simulink model "case5"  (R2024b)
settings: Solver=FixedStepAuto  StartTime=0  StopTime=1  FixedStep=1e-7  RelTol=1e-3
values from neighbouring files (symbols this model uses):
  SG_D_1_D = 0.01056    [IEEE9_case_parameters.m]    (also in case1_parameters.m; case2_parameters.m; case3_parameters.m; case4_parameters.m)
  SG_D_1_EnableSaturation = 0    [IEEE9_case_parameters.m]    (also in case1_parameters.m; case2_parameters.m; case3_parameters.m; case4_parameters.m)
  SG_D_1_f0 = 60    [IEEE9_case_parameters.m]    (also in case1_parameters.m; case2_parameters.m; case3_parameters.m; case4_parameters.m)
  SG_D_1_H = 7.5    [IEEE9_case_parameters.m]    (also in case1_parameters.m; case2_parameters.m; case3_parameters.m; case4_parameters.m)
  SG_D_1_K_A = 20    [IEEE9_case_parameters.m]    (also in case1_parameters.m; case2_parameters.m; case3_parameters.m; case4_parameters.m)
  SG_D_1_K_E = 1.000000e+1    (= 10)    [IEEE9_case_parameters.m]    (also in case1_parameters.m; case2_parameters.m; case3_parameters.m; case4_parameters.m)
  SG_D_1_K_F = 2.363    [IEEE9_case_parameters.m]    (also in case1_parameters.m; case2_parameters.m; case3_parameters.m; case4_parameters.m)
  SG_D_1_K_s = 0.5    [IEEE9_case_parameters.m]    (also in case1_parameters.m = 5; case2_parameters.m = 5; case3_parameters.m = 5; case4_parameters.m = 5)
  SG_D_1_R_a = 0.001088    [IEEE9_case_parameters.m]    (also in case1_parameters.m; case2_parameters.m; case3_parameters.m; case4_parameters.m)
  SG_D_1_S_A = 1    [IEEE9_case_parameters.m]    (also in case1_parameters.m; case2_parameters.m; case3_parameters.m; case4_parameters.m)
  SG_D_1_S_B = 0.103    [IEEE9_case_parameters.m]    (also in case1_parameters.m; case2_parameters.m; case3_parameters.m; case4_parameters.m)
  SG_D_1_S_N = 10.659857    [IEEE9_case_parameters.m]    (also in case1_parameters.m; case2_parameters.m; case3_parameters.m; case4_parameters.m)
  SG_D_1_SpeedPara = 200    [IEEE9_case_parameters.m]    (also in case1_parameters.m; case2_parameters.m; case3_parameters.m; case4_parameters.m)
  SG_D_1_T_0 = 0.720173    [IEEE9_case_parameters.m]    (also in case1_parameters.m = 0.755522; case2_parameters.m = 0.808931; case3_parameters.m = 0.869402; case4_parameters.m = 0.729316)
  SG_D_1_T_1 = 0.3    [IEEE9_case_parameters.m]    (also in case1_parameters.m; case2_parameters.m; case3_parameters.m; case4_parameters.m)
  SG_D_1_T_2 = 0.05    [IEEE9_case_parameters.m]    (also in case1_parameters.m; case2_parameters.m; case3_parameters.m; case4_parameters.m)
  SG_D_1_T_3 = 0.02    [IEEE9_case_parameters.m]    (also in case1_parameters.m; case2_parameters.m; case3_parameters.m; case4_parameters.m)
  SG_D_1_T_4 = 0.005    [IEEE9_case_parameters.m]    (also in case1_parameters.m; case2_parameters.m; case3_parameters.m; case4_parameters.m)
  SG_D_1_T_A = 0.02    [IEEE9_case_parameters.m]    (also in case1_parameters.m; case2_parameters.m; case3_parameters.m; case4_parameters.m)
  SG_D_1_T_dd = 8.000000e+0    (= 8)    [IEEE9_case_parameters.m]    (also in case1_parameters.m; case2_parameters.m; case3_parameters.m; case4_parameters.m)
  SG_D_1_T_ddd = 0.04    [IEEE9_case_parameters.m]    (also in case1_parameters.m; case2_parameters.m; case3_parameters.m; case4_parameters.m)
  SG_D_1_T_E = 0.314    [IEEE9_case_parameters.m]    (also in case1_parameters.m; case2_parameters.m; case3_parameters.m; case4_parameters.m)
  SG_D_1_T_F = 0.35    [IEEE9_case_parameters.m]    (also in case1_parameters.m; case2_parameters.m; case3_parameters.m; case4_parameters.m)
  SG_D_1_T_qd = 0.8    [IEEE9_case_parameters.m]    (also in case1_parameters.m; case2_parameters.m; case3_parameters.m; case4_parameters.m)
  SG_D_1_T_qdd = 0.02    [IEEE9_case_parameters.m]    (also in case1_parameters.m; case2_parameters.m; case3_parameters.m; case4_parameters.m)
  SG_D_1_T_speed = 0.1    [IEEE9_case_parameters.m]    (also in case1_parameters.m = 200; case2_parameters.m = 200; case3_parameters.m = 200; case4_parameters.m = 200)
  SG_D_1_T_w = 0.5    [IEEE9_case_parameters.m]    (also in case1_parameters.m; case2_parameters.m; case3_parameters.m; case4_parameters.m)
  SG_D_1_V_ref = 1.990276    [IEEE9_case_parameters.m]    (also in case1_parameters.m = 2.042296; case2_parameters.m = 2.051388; case3_parameters.m = 2.089584; case4_parameters.m = 2.01845)
  SG_D_1_w_ref = 376.991118    [IEEE9_case_parameters.m]    (also in case1_parameters.m; case2_parameters.m; case3_parameters.m; case4_parameters.m)
  SG_D_1_wb = 6.000000e+1    (= 60)    [IEEE9_case_parameters.m]    (also in case1_parameters.m; case2_parameters.m; case3_parameters.m; case4_parameters.m)
  SG_D_1_x_d = 1.9    [IEEE9_case_parameters.m]    (also in case1_parameters.m; case2_parameters.m; case3_parameters.m; case4_parameters.m)
  SG_D_1_x_dd = 0.302    [IEEE9_case_parameters.m]    (also in case1_parameters.m; case2_parameters.m; case3_parameters.m; case4_parameters.m)
  SG_D_1_x_ddd = 0.204    [IEEE9_case_parameters.m]    (also in case1_parameters.m; case2_parameters.m; case3_parameters.m; case4_parameters.m)
  SG_D_1_x_l = 0.05    [IEEE9_case_parameters.m]    (also in case1_parameters.m; case2_parameters.m; case3_parameters.m; case4_parameters.m)
  SG_D_1_x_q = 1.3    [IEEE9_case_parameters.m]    (also in case1_parameters.m; case2_parameters.m; case3_parameters.m; case4_parameters.m)
  SG_D_1_x_qd = 0.5    [IEEE9_case_parameters.m]    (also in case1_parameters.m; case2_parameters.m; case3_parameters.m; case4_parameters.m)
  SG_D_1_x_qdd = 0.3    [IEEE9_case_parameters.m]    (also in case1_parameters.m; case2_parameters.m; case3_parameters.m; case4_parameters.m)
  SG_D_2_D = 0.02    [IEEE9_case_parameters.m]    (also in case1_parameters.m; case2_parameters.m; case3_parameters.m; case4_parameters.m)
  SG_D_2_EnableSaturation = 0    [IEEE9_case_parameters.m]    (also in case1_parameters.m; case2_parameters.m; case3_parameters.m; case4_parameters.m)
  SG_D_2_f0 = 60    [IEEE9_case_parameters.m]    (also in case1_parameters.m; case2_parameters.m; case3_parameters.m; case4_parameters.m)
  SG_D_2_H = 8.000000e+0    (= 8)    [IEEE9_case_parameters.m]    (also in case1_parameters.m; case2_parameters.m; case3_parameters.m; case4_parameters.m)
  SG_D_2_K_A = 20    [IEEE9_case_parameters.m]    (also in case1_parameters.m; case2_parameters.m; case3_parameters.m; case4_parameters.m)
  SG_D_2_K_E = 1.000000e+1    (= 10)    [IEEE9_case_parameters.m]    (also in case1_parameters.m; case2_parameters.m; case3_parameters.m; case4_parameters.m)
  SG_D_2_K_F = 2.363    [IEEE9_case_parameters.m]    (also in case1_parameters.m; case2_parameters.m; case3_parameters.m; case4_parameters.m)
  SG_D_2_K_s = 0.5    [IEEE9_case_parameters.m]    (also in case1_parameters.m = 4; case2_parameters.m = 4; case3_parameters.m = 4; case4_parameters.m = 4)
  SG_D_2_R_a = 0.001088    [IEEE9_case_parameters.m]    (also in case1_parameters.m; case2_parameters.m; case3_parameters.m; case4_parameters.m)
  SG_D_2_S_A = 1    [IEEE9_case_parameters.m]    (also in case1_parameters.m; case2_parameters.m; case3_parameters.m; case4_parameters.m)
  SG_D_2_S_B = 0.103    [IEEE9_case_parameters.m]    (also in case1_parameters.m; case2_parameters.m; case3_parameters.m; case4_parameters.m)
  SG_D_2_S_N = 10.659857    [IEEE9_case_parameters.m]    (also in case1_parameters.m; case2_parameters.m; case3_parameters.m; case4_parameters.m)
  SG_D_2_SpeedPara = 200    [IEEE9_case_parameters.m]    (also in case1_parameters.m; case2_parameters.m; case3_parameters.m; case4_parameters.m)
  SG_D_2_T_0 = 1.632913    [IEEE9_case_parameters.m]    (also in case1_parameters.m = 1.632925; case2_parameters.m = 1.632915; case3_parameters.m = 1.632914; case4_parameters.m = 1.632927)
  SG_D_2_T_1 = 0.2    [IEEE9_case_parameters.m]    (also in case1_parameters.m; case2_parameters.m; case3_parameters.m; case4_parameters.m)
  SG_D_2_T_2 = 0.05    [IEEE9_case_parameters.m]    (also in case1_parameters.m; case2_parameters.m; case3_parameters.m; case4_parameters.m)
  SG_D_2_T_3 = 0.02    [IEEE9_case_parameters.m]    (also in case1_parameters.m; case2_parameters.m; case3_parameters.m; case4_parameters.m)
  SG_D_2_T_4 = 0.005    [IEEE9_case_parameters.m]    (also in case1_parameters.m; case2_parameters.m; case3_parameters.m; case4_parameters.m)
  SG_D_2_T_A = 0.02    [IEEE9_case_parameters.m]    (also in case1_parameters.m; case2_parameters.m; case3_parameters.m; case4_parameters.m)
  SG_D_2_T_dd = 7.9    [IEEE9_case_parameters.m]    (also in case1_parameters.m; case2_parameters.m; case3_parameters.m; case4_parameters.m)
  SG_D_2_T_ddd = 0.04    [IEEE9_case_parameters.m]    (also in case1_parameters.m; case2_parameters.m; case3_parameters.m; case4_parameters.m)
  SG_D_2_T_E = 0.314    [IEEE9_case_parameters.m]    (also in case1_parameters.m; case2_parameters.m; case3_parameters.m; case4_parameters.m)
  SG_D_2_T_F = 0.35    [IEEE9_case_parameters.m]    (also in case1_parameters.m; case2_parameters.m; case3_parameters.m; case4_parameters.m)
  SG_D_2_T_qd = 0.8    [IEEE9_case_parameters.m]    (also in case1_parameters.m; case2_parameters.m; case3_parameters.m; case4_parameters.m)
  SG_D_2_T_qdd = 0.015    [IEEE9_case_parameters.m]    (also in case1_parameters.m; case2_parameters.m; case3_parameters.m; case4_parameters.m)
  SG_D_2_T_speed = 0.1    [IEEE9_case_parameters.m]    (also in case1_parameters.m = 150; case2_parameters.m = 150; case3_parameters.m = 150; case4_parameters.m = 150)
  SG_D_2_T_w = 0.35    [IEEE9_case_parameters.m]    (also in case1_parameters.m; case2_parameters.m; case3_parameters.m; case4_parameters.m)
  SG_D_2_V_ref = 2.58547    [IEEE9_case_parameters.m]    (also in case1_parameters.m = 2.597896; case2_parameters.m = 2.587136; case3_parameters.m = 2.586042; case4_parameters.m = 2.599679)
  SG_D_2_w_ref = 376.991118    [IEEE9_case_parameters.m]    (also in case1_parameters.m; case2_parameters.m; case3_parameters.m; case4_parameters.m)
  SG_D_2_wb = 6.000000e+1    (= 60)    [IEEE9_case_parameters.m]    (also in case1_parameters.m; case2_parameters.m; case3_parameters.m; case4_parameters.m)
  SG_D_2_x_d = 1.8    [IEEE9_case_parameters.m]    (also in case1_parameters.m; case2_parameters.m; case3_parameters.m; case4_parameters.m)
  SG_D_2_x_dd = 0.302    [IEEE9_case_parameters.m]    (also in case1_parameters.m; case2_parameters.m; case3_parameters.m; case4_parameters.m)
  SG_D_2_x_ddd = 0.204    [IEEE9_case_parameters.m]    (also in case1_parameters.m; case2_parameters.m; case3_parameters.m; case4_parameters.m)
  SG_D_2_x_l = 0.05    [IEEE9_case_parameters.m]    (also in case1_parameters.m; case2_parameters.m; case3_parameters.m; case4_parameters.m)
  SG_D_2_x_q = 1.25    [IEEE9_case_parameters.m]    (also in case1_parameters.m; case2_parameters.m; case3_parameters.m; case4_parameters.m)
  SG_D_2_x_qd = 0.5    [IEEE9_case_parameters.m]    (also in case1_parameters.m; case2_parameters.m; case3_parameters.m; case4_parameters.m)
  SG_D_2_x_qdd = 0.3    [IEEE9_case_parameters.m]    (also in case1_parameters.m; case2_parameters.m; case3_parameters.m; case4_parameters.m)
  SG_D_3_D = 0.02    [IEEE9_case_parameters.m]    (also in case1_parameters.m; case2_parameters.m; case3_parameters.m; case4_parameters.m)
  SG_D_3_EnableSaturation = 0    [IEEE9_case_parameters.m]    (also in case1_parameters.m; case2_parameters.m; case3_parameters.m; case4_parameters.m)
  SG_D_3_f0 = 60    [IEEE9_case_parameters.m]    (also in case1_parameters.m; case2_parameters.m; case3_parameters.m; case4_parameters.m)
  SG_D_3_H = 7.7    [IEEE9_case_parameters.m]    (also in case1_parameters.m; case2_parameters.m; case3_parameters.m; case4_parameters.m)
  SG_D_3_K_A = 20    [IEEE9_case_parameters.m]    (also in case1_parameters.m; case2_parameters.m; case3_parameters.m; case4_parameters.m)
  SG_D_3_K_E = 1.000000e+1    (= 10)    [IEEE9_case_parameters.m]    (also in case1_parameters.m; case2_parameters.m; case3_parameters.m; case4_parameters.m)
  SG_D_3_K_F = 2.363    [IEEE9_case_parameters.m]    (also in case1_parameters.m; case2_parameters.m; case3_parameters.m; case4_parameters.m)
  SG_D_3_K_s = 0.2    [IEEE9_case_parameters.m]    (also in case1_parameters.m = 2; case2_parameters.m = 2; case3_parameters.m = 2; case4_parameters.m = 2)
  SG_D_3_R_a = 0.001088    [IEEE9_case_parameters.m]    (also in case1_parameters.m; case2_parameters.m; case3_parameters.m; case4_parameters.m)
  SG_D_3_S_A = 1    [IEEE9_case_parameters.m]    (also in case1_parameters.m; case2_parameters.m; case3_parameters.m; case4_parameters.m)
  SG_D_3_S_B = 0.103    [IEEE9_case_parameters.m]    (also in case1_parameters.m; case2_parameters.m; case3_parameters.m; case4_parameters.m)
  SG_D_3_S_N = 10.659857    [IEEE9_case_parameters.m]    (also in case1_parameters.m; case2_parameters.m; case3_parameters.m; case4_parameters.m)
  SG_D_3_SpeedPara = 200    [IEEE9_case_parameters.m]    (also in case1_parameters.m; case2_parameters.m; case3_parameters.m; case4_parameters.m)
  SG_D_3_T_0 = 0.850788    [IEEE9_case_parameters.m]    (also in case1_parameters.m = 0.850786; case2_parameters.m = 0.850787; case3_parameters.m; case4_parameters.m = 0.850786)
  SG_D_3_T_1 = 0.2    [IEEE9_case_parameters.m]    (also in case1_parameters.m; case2_parameters.m; case3_parameters.m; case4_parameters.m)
  SG_D_3_T_2 = 0.05    [IEEE9_case_parameters.m]    (also in case1_parameters.m; case2_parameters.m; case3_parameters.m; case4_parameters.m)
  SG_D_3_T_3 = 0.02    [IEEE9_case_parameters.m]    (also in case1_parameters.m; case2_parameters.m; case3_parameters.m; case4_parameters.m)
  SG_D_3_T_4 = 0.005    [IEEE9_case_parameters.m]    (also in case1_parameters.m; case2_parameters.m; case3_parameters.m; case4_parameters.m)
  SG_D_3_T_A = 0.02    [IEEE9_case_parameters.m]    (also in case1_parameters.m; case2_parameters.m; case3_parameters.m; case4_parameters.m)
  SG_D_3_T_dd = 8.1    [IEEE9_case_parameters.m]    (also in case1_parameters.m; case2_parameters.m; case3_parameters.m; case4_parameters.m)
  SG_D_3_T_ddd = 0.04    [IEEE9_case_parameters.m]    (also in case1_parameters.m; case2_parameters.m; case3_parameters.m; case4_parameters.m)
  SG_D_3_T_E = 0.314    [IEEE9_case_parameters.m]    (also in case1_parameters.m; case2_parameters.m; case3_parameters.m; case4_parameters.m)
  SG_D_3_T_F = 0.35    [IEEE9_case_parameters.m]    (also in case1_parameters.m; case2_parameters.m; case3_parameters.m; case4_parameters.m)
  SG_D_3_T_qd = 0.8    [IEEE9_case_parameters.m]    (also in case1_parameters.m; case2_parameters.m; case3_parameters.m; case4_parameters.m)
  SG_D_3_T_qdd = 0.015    [IEEE9_case_parameters.m]    (also in case1_parameters.m; case2_parameters.m; case3_parameters.m; case4_parameters.m)
  SG_D_3_T_speed = 0.1    [IEEE9_case_parameters.m]    (also in case1_parameters.m = 180; case2_parameters.m = 180; case3_parameters.m = 180; case4_parameters.m = 180)
  SG_D_3_T_w = 0.4    [IEEE9_case_parameters.m]    (also in case1_parameters.m; case2_parameters.m; case3_parameters.m; case4_parameters.m)
  SG_D_3_V_ref = 1.892727    [IEEE9_case_parameters.m]    (also in case1_parameters.m = 1.906439; case2_parameters.m = 1.895535; case3_parameters.m = 1.892105; case4_parameters.m = 1.906598)
  SG_D_3_w_ref = 376.991118    [IEEE9_case_parameters.m]    (also in case1_parameters.m; case2_parameters.m; case3_parameters.m; case4_parameters.m)
  SG_D_3_wb = 6.000000e+1    (= 60)    [IEEE9_case_parameters.m]    (also in case1_parameters.m; case2_parameters.m; case3_parameters.m; case4_parameters.m)
  SG_D_3_x_d = 1.85    [IEEE9_case_parameters.m]    (also in case1_parameters.m; case2_parameters.m; case3_parameters.m; case4_parameters.m)
  SG_D_3_x_dd = 0.302    [IEEE9_case_parameters.m]    (also in case1_parameters.m; case2_parameters.m; case3_parameters.m; case4_parameters.m)
  SG_D_3_x_ddd = 0.204    [IEEE9_case_parameters.m]    (also in case1_parameters.m; case2_parameters.m; case3_parameters.m; case4_parameters.m)
  SG_D_3_x_l = 0.05    [IEEE9_case_parameters.m]    (also in case1_parameters.m; case2_parameters.m; case3_parameters.m; case4_parameters.m)
  SG_D_3_x_q = 1.2    [IEEE9_case_parameters.m]    (also in case1_parameters.m; case2_parameters.m; case3_parameters.m; case4_parameters.m)
  SG_D_3_x_qd = 0.5    [IEEE9_case_parameters.m]    (also in case1_parameters.m; case2_parameters.m; case3_parameters.m; case4_parameters.m)
  SG_D_3_x_qdd = 0.3    [IEEE9_case_parameters.m]    (also in case1_parameters.m; case2_parameters.m; case3_parameters.m; case4_parameters.m)
(part 9 of 12)

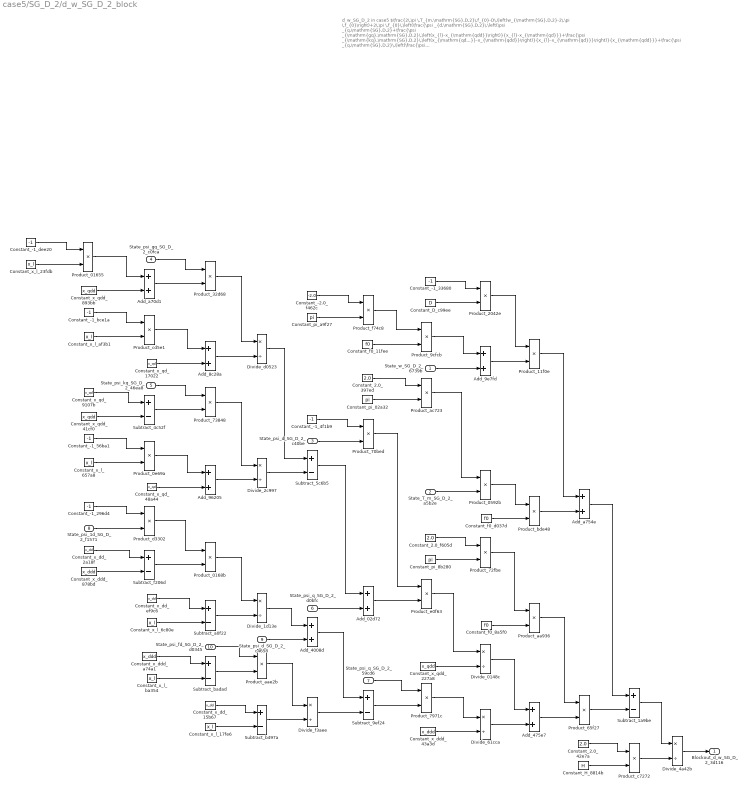
== system case5/SG_D_2/d_w_SG_D_2_block ==
  note: d_w_SG_D_2 in case5
      | $\frac{2\,\pi \,T_{m,\mathrm{SG},D,2}\,f_{0}-D\,\left(w_{\mathrm{SG},D,2}-2\,\pi \,f_{0}\right)+2\,\pi \,f_{0}\,\left(\frac{\psi _{d,\mathrm{SG},D,2}\,\left(\psi _{q,\mathrm{SG},D,2}+\frac{\psi _{\mathrm{gq},\mathrm{SG},D,2}\,\left(x_{l}-x_{\mathrm{qdd}}\right)}{x_{l}-x_{\mathrm{qd}}}+\frac{\psi _{\mathrm{kq},\mathrm{SG},D,2}\,\left(x_{\mathrm{qd}}-x_{\mathrm{qdd}}\right)}{x_{l}-x_{\mathrm{qd}}}\right)}{x_{\mathrm{qdd}}}+\frac{\psi _{q,\mathrm{SG},D,2}\,\left(\frac{\psi _{\mathrm{1d},\mathrm{SG},D,2}\,\left(x_{\mathrm{dd}}-x_{\mathrm{ddd}}\right)}{x_{\mathrm{dd}}-x_{l}}-\psi _{d,\mathrm{SG},D,2}+\frac{\psi _{\mathrm{fd},\mathrm{SG},D,2}\,\left(x_{\mathrm{ddd}}-x_{l}\right)}{x_{\mathrm{dd}}-x_{l}}\right)}{x_{\mathrm{ddd}}}\right)}{2\,H}$
      | Automatically generated on 2025-10-31 19:11:25 .
  State_w_SG_D_2_6739b : Inport
  State_T_m_SG_D_2_a5b2e : Inport  Port=2
  State_psi_d_SG_D_2_c40be : Inport  Port=3
  State_psi_gq_SG_D_2_c0fca : Inport  Port=4
  State_psi_kq_SG_D_2_46ea8 : Inport  Port=5
  State_psi_q_SG_D_2_d0bfc : Inport  Port=6
  State_psi_q_SG_D_2_59cd6 : Inport  Port=7
  State_psi_1d_SG_D_2_f1571 : Inport  Port=8
  State_psi_d_SG_D_2_c4658 : Inport  Port=9
  State_psi_fd_SG_D_2_d0345 : Inport  Port=10
  Add_02d72 : Sum
  Add_4008d : Sum
  Add_475e7 : Sum
  Add_8c28a : Sum
  Add_96205 : Sum
  Add_9e7fd : Sum
  Add_a70d1 : Sum
  Add_a754e : Sum
  Constant_-1_296d4 : Constant  Value=-1
  Constant_-1_33680 : Constant  Value=-1
  Constant_-1_4f1b9 : Constant  Value=-1
  Constant_-1_56ba1 : Constant  Value=-1
  Constant_-1_bce1a : Constant  Value=-1
  Constant_-1_dee20 : Constant  Value=-1
  Constant_-2.0_f462c : Constant  Value=-2.0
  Constant_2.0_397ed : Constant  Value=2.0
  Constant_2.0_42e7a : Constant  Value=2.0
  Constant_2.0_f605d : Constant  Value=2.0
  Constant_D_c99ee : Constant  Value=D
  Constant_H_8814b : Constant  Value=H
  Constant_f0_11fee : Constant  Value=f0
  Constant_f0_8a5f0 : Constant  Value=f0
  Constant_f0_d037d : Constant  Value=f0
  Constant_pi_02a32 : Constant  Value=pi
  Constant_pi_8b280 : Constant  Value=pi
  Constant_pi_a9f27 : Constant  Value=pi
  Constant_x_dd_15b67 : Constant  Value=x_dd
  Constant_x_dd_2a18f : Constant  Value=x_dd
  Constant_x_dd_ef9c6 : Constant  Value=x_dd
  Constant_x_ddd_43a3d : Constant  Value=x_ddd
  Constant_x_ddd_878bd : Constant  Value=x_ddd
  Constant_x_ddd_a74a1 : Constant  Value=x_ddd
  Constant_x_l_17fe6 : Constant  Value=x_l
  Constant_x_l_23fdb : Constant  Value=x_l
  Constant_x_l_657a8 : Constant  Value=x_l
  Constant_x_l_6c80e : Constant  Value=x_l
  Constant_x_l_af3b1 : Constant  Value=x_l
  Constant_x_l_ba354 : Constant  Value=x_l
  Constant_x_qd_17022 : Constant  Value=x_qd
  Constant_x_qd_48a44 : Constant  Value=x_qd
  Constant_x_qd_9107b : Constant  Value=x_qd
  Constant_x_qdd_227a8 : Constant  Value=x_qdd
  Constant_x_qdd_41cf0 : Constant  Value=x_qdd
  Constant_x_qdd_893bb : Constant  Value=x_qdd
  Divide_0148c : Product  Inputs=*/
  Divide_1d13e : Product  Inputs=*/
  Divide_2c997 : Product  Inputs=*/
  Divide_4a42b : Product  Inputs=*/
  Divide_61cca : Product  Inputs=*/
  Divide_d0523 : Product  Inputs=*/
  Divide_f3aee : Product  Inputs=*/
  Product_01655 : Product
  Product_0168b : Product
  Product_0592b : Product
  Product_0e69a : Product
  Product_11f0e : Product
  Product_2042e : Product
  Product_32d68 : Product
  Product_65f27 : Product
  Product_70bed : Product
  Product_72fbe : Product
  Product_73848 : Product
  Product_7971c : Product
  Product_9cfcb : Product
  Product_aa936 : Product
  Product_aae2b : Product
  Product_ac723 : Product
  Product_bde48 : Product
  Product_c7272 : Product
  Product_cd5e1 : Product
  Product_d3302 : Product
  Product_e0f63 : Product
  Product_f74c8 : Product
  Subtract_1a9be : Sum  Inputs=+-
  Subtract_4c52f : Sum  Inputs=+-
  Subtract_5c6b5 : Sum  Inputs=+-
  Subtract_9ef24 : Sum  Inputs=+-
  Subtract_a0f22 : Sum  Inputs=+-
  Subtract_b497a : Sum  Inputs=+-
  Subtract_badad : Sum  Inputs=+-
  Subtract_f206d : Sum  Inputs=+-
  Blockout_d_w_SG_D_2_3d116 : Outport
  wires:
  Constant_x_qd_9107b/1 -> Subtract_4c52f/1
  Constant_-1_56ba1/1 -> Product_0e69a/1
  Constant_-1_dee20/1 -> Product_01655/1
  Constant_x_qdd_41cf0/1 -> Subtract_4c52f/2
  Subtract_b497a/1 -> Divide_f3aee/2
  Constant_x_l_657a8/1 -> Product_0e69a/2
  Constant_x_l_23fdb/1 -> Product_01655/2
  Product_0e69a/1 -> Add_96205/1
  Product_01655/1 -> Add_a70d1/1
  Constant_x_l_6c80e/1 -> Subtract_a0f22/2
  Constant_x_l_af3b1/1 -> Product_cd5e1/2
  Constant_x_ddd_43a3d/1 -> Divide_61cca/2
  Subtract_badad/1 -> Product_aae2b/2
  Constant_x_qd_48a44/1 -> Add_96205/2
  Constant_x_qdd_893bb/1 -> Add_a70d1/2
  Constant_-1_bce1a/1 -> Product_cd5e1/1
  State_psi_d_SG_D_2_c40be/1 -> Product_70bed/2
  Constant_-1_296d4/1 -> Product_d3302/1
  State_w_SG_D_2_6739b/1 -> Add_9e7fd/2
  Product_cd5e1/1 -> Add_8c28a/1
  State_psi_1d_SG_D_2_f1571/1 -> Product_d3302/2
  Constant_x_dd_2a18f/1 -> Subtract_f206d/1
  Divide_d0523/1 -> Subtract_5c6b5/1
  Subtract_4c52f/1 -> Product_73848/2
  Constant_x_ddd_878bd/1 -> Subtract_f206d/2
  State_psi_gq_SG_D_2_c0fca/1 -> Product_32d68/1
  Add_96205/1 -> Divide_2c997/2
  State_psi_d_SG_D_2_c4658/1 -> Add_4008d/2
  Add_a70d1/1 -> Product_32d68/2
  Constant_x_qd_17022/1 -> Add_8c28a/2
  State_psi_kq_SG_D_2_46ea8/1 -> Product_73848/1
  Product_d3302/1 -> Product_0168b/1
  Subtract_f206d/1 -> Product_0168b/2
  Constant_pi_02a32/1 -> Product_ac723/2
  Constant_x_dd_ef9c6/1 -> Subtract_a0f22/1
  Constant_x_ddd_a74a1/1 -> Subtract_badad/1
  Constant_x_l_ba354/1 -> Subtract_badad/2
  Product_32d68/1 -> Divide_d0523/1
  Add_8c28a/1 -> Divide_d0523/2
  Add_02d72/1 -> Product_e0f63/2
  Product_73848/1 -> Divide_2c997/1
  Constant_pi_a9f27/1 -> Product_f74c8/2
  Product_0168b/1 -> Divide_1d13e/1
  Subtract_a0f22/1 -> Divide_1d13e/2
  State_psi_fd_SG_D_2_d0345/1 -> Product_aae2b/1
  Divide_1d13e/1 -> Add_4008d/1
  Constant_x_dd_15b67/1 -> Subtract_b497a/1
  Constant_x_l_17fe6/1 -> Subtract_b497a/2
  Divide_2c997/1 -> Subtract_5c6b5/2
  Product_aae2b/1 -> Divide_f3aee/1
  Constant_-1_4f1b9/1 -> Product_70bed/1
  Constant_-2.0_f462c/1 -> Product_f74c8/1
  Subtract_5c6b5/1 -> Add_02d72/1
  Subtract_9ef24/1 -> Product_7971c/2
  State_psi_q_SG_D_2_d0bfc/1 -> Add_02d72/2
  Constant_D_c99ee/1 -> Product_2042e/2
  Add_4008d/1 -> Subtract_9ef24/1
  Divide_f3aee/1 -> Subtract_9ef24/2
  Product_f74c8/1 -> Product_9cfcb/1
  Constant_f0_11fee/1 -> Product_9cfcb/2
  Constant_2.0_397ed/1 -> Product_ac723/1
  Product_70bed/1 -> Product_e0f63/1
  State_psi_q_SG_D_2_59cd6/1 -> Product_7971c/1
  Constant_-1_33680/1 -> Product_2042e/1
  Product_9cfcb/1 -> Add_9e7fd/1
  Product_ac723/1 -> Product_0592b/1
  State_T_m_SG_D_2_a5b2e/1 -> Product_0592b/2
  Constant_2.0_f605d/1 -> Product_72fbe/1
  Constant_pi_8b280/1 -> Product_72fbe/2
  Product_e0f63/1 -> Divide_0148c/1
  Constant_x_qdd_227a8/1 -> Divide_0148c/2
  Product_7971c/1 -> Divide_61cca/1
  Product_2042e/1 -> Product_11f0e/1
  Add_9e7fd/1 -> Product_11f0e/2
  Product_0592b/1 -> Product_bde48/1
  Constant_f0_d037d/1 -> Product_bde48/2
  Product_72fbe/1 -> Product_aa936/1
  Constant_f0_8a5f0/1 -> Product_aa936/2
  Divide_0148c/1 -> Add_475e7/1
  Divide_61cca/1 -> Add_475e7/2
  Product_11f0e/1 -> Add_a754e/1
  Product_bde48/1 -> Add_a754e/2
  Product_aa936/1 -> Product_65f27/1
  Add_475e7/1 -> Product_65f27/2
  Add_a754e/1 -> Subtract_1a9be/1
  Product_65f27/1 -> Subtract_1a9be/2
  Constant_2.0_42e7a/1 -> Product_c7272/1
  Constant_H_8814b/1 -> Product_c7272/2
  Subtract_1a9be/1 -> Divide_4a42b/1
  Product_c7272/1 -> Divide_4a42b/2
  Divide_4a42b/1 -> Blockout_d_w_SG_D_2_3d116/1

== system case5/SG_D_2/i_d_SG_D_2_block ==
  note: i_d_SG_D_2 in case5
      | $\frac{\sin\left(\theta _{\mathrm{SG},D,2}\right)\,\left(\frac{\psi _{\mathrm{1d},\mathrm{SG},D,2}\,\left(x_{\mathrm{dd}}-x_{\mathrm{ddd}}\right)}{x_{\mathrm{dd}}-x_{l}}-\psi _{d,\mathrm{SG},D,2}+\frac{\psi _{\mathrm{fd},\mathrm{SG},D,2}\,\left(x_{\mathrm{ddd}}-x_{l}\right)}{x_{\mathrm{dd}}-x_{l}}\right)}{x_{\mathrm{ddd}}}-\frac{\cos\left(\theta _{\mathrm{SG},D,2}\right)\,\left(\psi _{q,\mathrm{SG},D,2}+\frac{\psi _{\mathrm{gq},\mathrm{SG},D,2}\,\left(x_{l}-x_{\mathrm{qdd}}\right)}{x_{l}-x_{\mathrm{qd}}}+\frac{\psi _{\mathrm{kq},\mathrm{SG},D,2}\,\left(x_{\mathrm{qd}}-x_{\mathrm{qdd}}\right)}{x_{l}-x_{\mathrm{qd}}}\right)}{x_{\mathrm{qdd}}}$
      | Automatically generated on 2025-10-31 19:11:50 .
  State_psi_gq_SG_D_2_2f279 : Inport
  State_psi_kq_SG_D_2_3a555 : Inport  Port=2
  State_psi_q_SG_D_2_2fd58 : Inport  Port=3
  State_theta_SG_D_2_e2546 : Inport  Port=4
  State_psi_1d_SG_D_2_aa18d : Inport  Port=5
  State_psi_d_SG_D_2_3866e : Inport  Port=6
  State_psi_fd_SG_D_2_ae8c9 : Inport  Port=7
  State_theta_SG_D_2_a5f3d : Inport  Port=8
  Add_13915 : Sum
  Add_36676 : Sum
  Add_73ce3 : Sum
  Add_92234 : Sum
  Add_a8fb6 : Sum
  Constant_-1_03d4f : Constant  Value=-1
  Constant_-1_1051d : Constant  Value=-1
  Constant_-1_34799 : Constant  Value=-1
  Constant_-1_463ac : Constant  Value=-1
  Constant_-1_d167b : Constant  Value=-1
  Constant_x_dd_18187 : Constant  Value=x_dd
  Constant_x_dd_6a4fb : Constant  Value=x_dd
  Constant_x_dd_7e17e : Constant  Value=x_dd
  Constant_x_ddd_6b299 : Constant  Value=x_ddd
  Constant_x_ddd_a24af : Constant  Value=x_ddd
  Constant_x_ddd_eefe1 : Constant  Value=x_ddd
  Constant_x_l_0bd46 : Constant  Value=x_l
  Constant_x_l_3aa8e : Constant  Value=x_l
  Constant_x_l_3c94c : Constant  Value=x_l
  Constant_x_l_61363 : Constant  Value=x_l
  Constant_x_l_74230 : Constant  Value=x_l
  Constant_x_l_fed2c : Constant  Value=x_l
  Constant_x_qd_0ee76 : Constant  Value=x_qd
  Constant_x_qd_463c9 : Constant  Value=x_qd
  Constant_x_qd_862b7 : Constant  Value=x_qd
  Constant_x_qdd_76983 : Constant  Value=x_qdd
  Constant_x_qdd_876d4 : Constant  Value=x_qdd
  Constant_x_qdd_f0996 : Constant  Value=x_qdd
  Divide_0ee9e : Product  Inputs=*/
  Divide_69b90 : Product  Inputs=*/
  Divide_74453 : Product  Inputs=*/
  Divide_8e4df : Product  Inputs=*/
  Divide_bbe97 : Product  Inputs=*/
  Divide_c93c3 : Product  Inputs=*/
  MathFunc_cos_962a1 : Trigonometry  Operator=cos
  MathFunc_sin_f99f8 : Trigonometry
  Product_1a99e : Product
  Product_20384 : Product
  Product_2af6a : Product
  Product_3035b : Product
  Product_4622d : Product
  Product_8b4c4 : Product
  Product_ae53a : Product
  Product_b8ef8 : Product
  Product_c3166 : Product
  Product_dd6be : Product
  Product_de29b : Product
  Subtract_0f27b : Sum  Inputs=+-
  Subtract_0f980 : Sum  Inputs=+-
  Subtract_75a6d : Sum  Inputs=+-
  Subtract_7e2df : Sum  Inputs=+-
  Subtract_a6082 : Sum  Inputs=+-
  Subtract_b3680 : Sum  Inputs=+-
  Subtract_da268 : Sum  Inputs=+-
  Subtract_f974f : Sum  Inputs=+-
  Blockout_i_d_SG_D_2_72f47 : Outport
  wires:
  Constant_x_ddd_a24af/1 -> Subtract_75a6d/1
  Constant_x_qd_463c9/1 -> Subtract_b3680/1
  Constant_-1_1051d/1 -> Product_4622d/1
  Constant_-1_34799/1 -> Product_3035b/1
  Subtract_a6082/1 -> Blockout_i_d_SG_D_2_72f47/1
  Constant_x_qdd_f0996/1 -> Subtract_b3680/2
  Constant_x_l_3aa8e/1 -> Product_4622d/2
  Constant_x_l_fed2c/1 -> Product_3035b/2
  Product_4622d/1 -> Add_92234/1
  Product_3035b/1 -> Add_36676/1
  Constant_x_l_3c94c/1 -> Product_b8ef8/2
  Constant_x_qd_862b7/1 -> Add_92234/2
  Constant_x_qdd_876d4/1 -> Add_36676/2
  Constant_x_qdd_76983/1 -> Divide_0ee9e/2
  MathFunc_cos_962a1/1 -> Product_8b4c4/2
  Constant_-1_d167b/1 -> Product_b8ef8/1
  State_psi_gq_SG_D_2_2f279/1 -> Product_ae53a/1
  Subtract_75a6d/1 -> Product_20384/2
  Product_c3166/1 -> Product_dd6be/1
  Add_92234/1 -> Divide_69b90/2
  Add_36676/1 -> Product_ae53a/2
  Product_20384/1 -> Divide_74453/1
  Product_b8ef8/1 -> Add_13915/1
  Constant_x_qd_0ee76/1 -> Add_13915/2
  State_theta_SG_D_2_a5f3d/1 -> MathFunc_sin_f99f8/1
  State_psi_kq_SG_D_2_3a555/1 -> Product_1a99e/1
  Add_a8fb6/1 -> Subtract_7e2df/1
  Subtract_b3680/1 -> Product_1a99e/2
  Product_ae53a/1 -> Divide_c93c3/1
  Constant_-1_03d4f/1 -> Product_c3166/1
  State_psi_1d_SG_D_2_aa18d/1 -> Product_c3166/2
  State_psi_fd_SG_D_2_ae8c9/1 -> Product_20384/1
  Constant_x_dd_7e17e/1 -> Subtract_0f27b/1
  Product_dd6be/1 -> Divide_bbe97/1
  Constant_x_ddd_eefe1/1 -> Subtract_0f27b/2
  Divide_74453/1 -> Subtract_7e2df/2
  Add_13915/1 -> Divide_c93c3/2
  Product_2af6a/1 -> Divide_8e4df/1
  Product_1a99e/1 -> Divide_69b90/1
  Constant_-1_463ac/1 -> Product_de29b/1
  Subtract_da268/1 -> Divide_74453/2
  Subtract_0f27b/1 -> Product_dd6be/2
  Constant_x_dd_6a4fb/1 -> Subtract_0f980/1
  Subtract_7e2df/1 -> Product_2af6a/1
  Constant_x_l_61363/1 -> Subtract_0f980/2
  Constant_x_l_74230/1 -> Subtract_75a6d/2
  Divide_c93c3/1 -> Subtract_f974f/1
  Divide_8e4df/1 -> Subtract_a6082/2
  Divide_69b90/1 -> Subtract_f974f/2
  Subtract_0f980/1 -> Divide_bbe97/2
  Constant_x_dd_18187/1 -> Subtract_da268/1
  Divide_0ee9e/1 -> Subtract_a6082/1
  Constant_x_l_0bd46/1 -> Subtract_da268/2
  Subtract_f974f/1 -> Add_73ce3/1
  State_psi_q_SG_D_2_2fd58/1 -> Add_73ce3/2
  Constant_x_ddd_6b299/1 -> Divide_8e4df/2
  MathFunc_sin_f99f8/1 -> Product_2af6a/2
  Divide_bbe97/1 -> Add_a8fb6/1
  State_psi_d_SG_D_2_3866e/1 -> Add_a8fb6/2
  Add_73ce3/1 -> Product_de29b/2
  State_theta_SG_D_2_e2546/1 -> MathFunc_cos_962a1/1
  Product_de29b/1 -> Product_8b4c4/1
  Product_8b4c4/1 -> Divide_0ee9e/1

== system case5/SG_D_2/i_q_SG_D_2_block ==
  note: i_q_SG_D_2 in case5
      | $-\frac{\sin\left(\theta _{\mathrm{SG},D,2}\right)\,\left(\psi _{q,\mathrm{SG},D,2}+\frac{\psi _{\mathrm{gq},\mathrm{SG},D,2}\,\left(x_{l}-x_{\mathrm{qdd}}\right)}{x_{l}-x_{\mathrm{qd}}}+\frac{\psi _{\mathrm{kq},\mathrm{SG},D,2}\,\left(x_{\mathrm{qd}}-x_{\mathrm{qdd}}\right)}{x_{l}-x_{\mathrm{qd}}}\right)}{x_{\mathrm{qdd}}}-\frac{\cos\left(\theta _{\mathrm{SG},D,2}\right)\,\left(\frac{\psi _{\mathrm{1d},\mathrm{SG},D,2}\,\left(x_{\mathrm{dd}}-x_{\mathrm{ddd}}\right)}{x_{\mathrm{dd}}-x_{l}}-\psi _{d,\mathrm{SG},D,2}+\frac{\psi _{\mathrm{fd},\mathrm{SG},D,2}\,\left(x_{\mathrm{ddd}}-x_{l}\right)}{x_{\mathrm{dd}}-x_{l}}\right)}{x_{\mathrm{ddd}}}$
      | Automatically generated on 2025-10-31 19:11:55 .
  State_psi_gq_SG_D_2_27a63 : Inport
  State_psi_kq_SG_D_2_d20f4 : Inport  Port=2
  State_psi_q_SG_D_2_28683 : Inport  Port=3
  State_theta_SG_D_2_24bbd : Inport  Port=4
  State_psi_1d_SG_D_2_19eb0 : Inport  Port=5
  State_psi_d_SG_D_2_881d1 : Inport  Port=6
  State_psi_fd_SG_D_2_80ec4 : Inport  Port=7
  State_theta_SG_D_2_e7cf1 : Inport  Port=8
  Add_0fb23 : Sum
  Add_1f302 : Sum
  Add_cd755 : Sum
  Add_df081 : Sum
  Add_e2828 : Sum
  Add_f72a5 : Sum
  Constant_-1_09393 : Constant  Value=-1
  Constant_-1_18aec : Constant  Value=-1
  Constant_-1_3d470 : Constant  Value=-1
  Constant_-1_452c5 : Constant  Value=-1
  Constant_-1_fe808 : Constant  Value=-1
  Constant_x_dd_36be5 : Constant  Value=x_dd
  Constant_x_dd_57552 : Constant  Value=x_dd
  Constant_x_dd_93985 : Constant  Value=x_dd
  Constant_x_ddd_19be5 : Constant  Value=x_ddd
  Constant_x_ddd_447f7 : Constant  Value=x_ddd
  Constant_x_ddd_ce0ab : Constant  Value=x_ddd
  Constant_x_l_1cd57 : Constant  Value=x_l
  Constant_x_l_33280 : Constant  Value=x_l
  Constant_x_l_4ae26 : Constant  Value=x_l
  Constant_x_l_8b246 : Constant  Value=x_l
  Constant_x_l_b095c : Constant  Value=x_l
  Constant_x_l_bd247 : Constant  Value=x_l
  Constant_x_qd_0c1f9 : Constant  Value=x_qd
  Constant_x_qd_36607 : Constant  Value=x_qd
  Constant_x_qd_a0e73 : Constant  Value=x_qd
  Constant_x_qdd_523d7 : Constant  Value=x_qdd
  Constant_x_qdd_5b401 : Constant  Value=x_qdd
  Constant_x_qdd_b534f : Constant  Value=x_qdd
  Divide_29683 : Product  Inputs=*/
  Divide_2f6c7 : Product  Inputs=*/
  Divide_354c4 : Product  Inputs=*/
  Divide_47f60 : Product  Inputs=*/
  Divide_623f5 : Product  Inputs=*/
  Divide_b9659 : Product  Inputs=*/
  MathFunc_cos_d17a9 : Trigonometry  Operator=cos
  MathFunc_sin_6e4a1 : Trigonometry
  Product_1e166 : Product
  Product_35351 : Product
  Product_4861a : Product
  Product_60abc : Product
  Product_6680b : Product
  Product_6700b : Product
  Product_78db1 : Product
  Product_89e1b : Product
  Product_8a303 : Product
  Product_bec09 : Product
  Product_db8f2 : Product
  Subtract_09687 : Sum  Inputs=+-
  Subtract_20d2a : Sum  Inputs=+-
  Subtract_2a004 : Sum  Inputs=+-
  Subtract_348ae : Sum  Inputs=+-
  Subtract_5d93e : Sum  Inputs=+-
  Subtract_e5516 : Sum  Inputs=+-
  Subtract_fdede : Sum  Inputs=+-
  Blockout_i_q_SG_D_2_ddca7 : Outport
  wires:
  MathFunc_sin_6e4a1/1 -> Product_1e166/2
  Product_bec09/1 -> Product_1e166/1
  Constant_-1_3d470/1 -> Product_4861a/1
  Constant_-1_09393/1 -> Product_78db1/1
  Constant_x_l_4ae26/1 -> Product_4861a/2
  Product_4861a/1 -> Add_0fb23/1
  Subtract_e5516/1 -> Product_6700b/2
  Constant_x_qdd_5b401/1 -> Subtract_09687/2
  Constant_x_qdd_b534f/1 -> Add_0fb23/2
  Add_f72a5/1 -> Product_bec09/2
  Constant_x_l_b095c/1 -> Product_78db1/2
  Constant_x_qd_a0e73/1 -> Subtract_09687/1
  Constant_-1_18aec/1 -> Product_db8f2/1
  Constant_x_l_bd247/1 -> Product_db8f2/2
  State_psi_1d_SG_D_2_19eb0/1 -> Product_8a303/2
  State_psi_gq_SG_D_2_27a63/1 -> Product_6680b/1
  Add_0fb23/1 -> Product_6680b/2
  Product_78db1/1 -> Add_cd755/1
  Divide_29683/1 -> Add_df081/1
  Constant_x_qd_0c1f9/1 -> Add_cd755/2
  State_psi_kq_SG_D_2_d20f4/1 -> Product_89e1b/1
  Add_1f302/1 -> Subtract_20d2a/1
  Constant_x_ddd_ce0ab/1 -> Subtract_e5516/2
  Subtract_09687/1 -> Product_89e1b/2
  Product_db8f2/1 -> Add_e2828/1
  Constant_x_qd_36607/1 -> Add_e2828/2
  Constant_-1_fe808/1 -> Product_8a303/1
  Constant_x_l_33280/1 -> Subtract_2a004/2
  Constant_x_dd_57552/1 -> Subtract_e5516/1
  Product_6680b/1 -> Divide_623f5/1
  Divide_47f60/1 -> Subtract_20d2a/2
  Add_cd755/1 -> Divide_623f5/2
  Product_60abc/1 -> Divide_b9659/1
  Product_89e1b/1 -> Divide_354c4/1
  Constant_-1_452c5/1 -> Product_bec09/1
  Product_8a303/1 -> Product_6700b/1
  Add_e2828/1 -> Divide_354c4/2
  Constant_x_dd_93985/1 -> Subtract_348ae/1
  Subtract_20d2a/1 -> Product_60abc/1
  Subtract_fdede/1 -> Product_35351/2
  Constant_x_l_8b246/1 -> Subtract_348ae/2
  Constant_x_ddd_19be5/1 -> Subtract_fdede/1
  Constant_x_l_1cd57/1 -> Subtract_fdede/2
  Divide_623f5/1 -> Subtract_5d93e/1
  Divide_b9659/1 -> Add_df081/2
  Product_35351/1 -> Divide_47f60/1
  Divide_354c4/1 -> Subtract_5d93e/2
  Subtract_2a004/1 -> Divide_47f60/2
  Product_6700b/1 -> Divide_2f6c7/1
  Subtract_348ae/1 -> Divide_2f6c7/2
  Constant_x_qdd_523d7/1 -> Divide_29683/2
  State_psi_fd_SG_D_2_80ec4/1 -> Product_35351/1
  Constant_x_dd_36be5/1 -> Subtract_2a004/1
  Subtract_5d93e/1 -> Add_f72a5/1
  State_psi_q_SG_D_2_28683/1 -> Add_f72a5/2
  Constant_x_ddd_447f7/1 -> Divide_b9659/2
  Divide_2f6c7/1 -> Add_1f302/1
  State_psi_d_SG_D_2_881d1/1 -> Add_1f302/2
  State_theta_SG_D_2_24bbd/1 -> MathFunc_sin_6e4a1/1
  State_theta_SG_D_2_e7cf1/1 -> MathFunc_cos_d17a9/1
  MathFunc_cos_d17a9/1 -> Product_60abc/2
  Product_1e166/1 -> Divide_29683/1
  Add_df081/1 -> Blockout_i_q_SG_D_2_ddca7/1

== system case5/SG_D_2/theta_SG_D_2_out_block ==
  note: theta_SG_D_2_out in case5
      | $\theta _{\mathrm{SG},D,2}$
      | Automatically generated on 2025-10-31 19:12:01 .
  State_theta_SG_D_2_369d6 : Inport
  Blockout_theta_SG_D_2_out_abd77 : Outport
  wires:
  State_theta_SG_D_2_369d6/1 -> Blockout_theta_SG_D_2_out_abd77/1

== system case5/SG_D_2/w_SG_D_2_out_block ==
  note: w_SG_D_2_out in case5
      | $w_{\mathrm{SG},D,2}$
      | Automatically generated on 2025-10-31 19:12:00 .
  State_w_SG_D_2_5e653 : Inport
  Blockout_w_SG_D_2_out_edd03 : Outport
  wires:
  State_w_SG_D_2_5e653/1 -> Blockout_w_SG_D_2_out_edd03/1

== system case5/SG_D_3/T_e_SG_D_3_block ==
  note: T_e_SG_D_3 in case5
      | $-\frac{\psi _{d,\mathrm{SG},D,3}\,\left(\psi _{q,\mathrm{SG},D,3}+\frac{\psi _{\mathrm{gq},\mathrm{SG},D,3}\,\left(x_{l}-x_{\mathrm{qdd}}\right)}{x_{l}-x_{\mathrm{qd}}}+\frac{\psi _{\mathrm{kq},\mathrm{SG},D,3}\,\left(x_{\mathrm{qd}}-x_{\mathrm{qdd}}\right)}{x_{l}-x_{\mathrm{qd}}}\right)}{x_{\mathrm{qdd}}}-\frac{\psi _{q,\mathrm{SG},D,3}\,\left(\frac{\psi _{\mathrm{1d},\mathrm{SG},D,3}\,\left(x_{\mathrm{dd}}-x_{\mathrm{ddd}}\right)}{x_{\mathrm{dd}}-x_{l}}-\psi _{d,\mathrm{SG},D,3}+\frac{\psi _{\mathrm{fd},\mathrm{SG},D,3}\,\left(x_{\mathrm{ddd}}-x_{l}\right)}{x_{\mathrm{dd}}-x_{l}}\right)}{x_{\mathrm{ddd}}}$
      | Automatically generated on 2025-10-31 19:13:26 .
  State_psi_d_SG_D_3_0515e : Inport
  State_psi_gq_SG_D_3_1cc94 : Inport  Port=2
  State_psi_kq_SG_D_3_f2804 : Inport  Port=3
  State_psi_q_SG_D_3_52c06 : Inport  Port=4
  State_psi_q_SG_D_3_d7233 : Inport  Port=5
  State_psi_1d_SG_D_3_44396 : Inport  Port=6
  State_psi_d_SG_D_3_355d2 : Inport  Port=7
  State_psi_fd_SG_D_3_44178 : Inport  Port=8
  Add_38c6f : Sum
  Add_424ea : Sum
  Add_75f47 : Sum
  Add_c136d : Sum
  Add_c8d7c : Sum
  Add_d6943 : Sum
  Constant_-1_54cd6 : Constant  Value=-1
  Constant_-1_7e7e8 : Constant  Value=-1
  Constant_-1_a4931 : Constant  Value=-1
  Constant_-1_bafa8 : Constant  Value=-1
  Constant_-1_e3bfe : Constant  Value=-1
  Constant_x_dd_3fcde : Constant  Value=x_dd
  Constant_x_dd_9d528 : Constant  Value=x_dd
  Constant_x_dd_c5962 : Constant  Value=x_dd
  Constant_x_ddd_03e8c : Constant  Value=x_ddd
  Constant_x_ddd_f9c1b : Constant  Value=x_ddd
  Constant_x_ddd_fc21e : Constant  Value=x_ddd
  Constant_x_l_08c9e : Constant  Value=x_l
  Constant_x_l_1b50a : Constant  Value=x_l
  Constant_x_l_49bee : Constant  Value=x_l
  Constant_x_l_7e92c : Constant  Value=x_l
  Constant_x_l_c4f31 : Constant  Value=x_l
  Constant_x_l_d57e3 : Constant  Value=x_l
  Constant_x_qd_46c4d : Constant  Value=x_qd
  Constant_x_qd_5fe02 : Constant  Value=x_qd
  Constant_x_qd_d77c2 : Constant  Value=x_qd
  Constant_x_qdd_03902 : Constant  Value=x_qdd
  Constant_x_qdd_35d62 : Constant  Value=x_qdd
  Constant_x_qdd_7b39c : Constant  Value=x_qdd
  Divide_57be3 : Product  Inputs=*/
  Divide_5f4e1 : Product  Inputs=*/
  Divide_6a35a : Product  Inputs=*/
  Divide_7ca07 : Product  Inputs=*/
  Divide_a7e4b : Product  Inputs=*/
  Divide_bf5f0 : Product  Inputs=*/
  Product_033c4 : Product
  Product_06a99 : Product
  Product_0aa49 : Product
  Product_3c439 : Product
  Product_60f0d : Product
  Product_65876 : Product
  Product_6f939 : Product
  Product_8dcb6 : Product
  Product_ae869 : Product
  Product_f9b9c : Product
  Product_fb25b : Product
  Subtract_278eb : Sum  Inputs=+-
  Subtract_3acb7 : Sum  Inputs=+-
  Subtract_5e39d : Sum  Inputs=+-
  Subtract_64596 : Sum  Inputs=+-
  Subtract_96906 : Sum  Inputs=+-
  Subtract_bf7b9 : Sum  Inputs=+-
  Subtract_ff6a0 : Sum  Inputs=+-
  Blockout_T_e_SG_D_3_5900b : Outport
  wires:
  State_psi_q_SG_D_3_52c06/1 -> Add_c136d/2
  Constant_-1_a4931/1 -> Product_8dcb6/1
  Subtract_96906/1 -> Product_033c4/2
  State_psi_1d_SG_D_3_44396/1 -> Product_f9b9c/2
  Constant_-1_7e7e8/1 -> Product_3c439/1
  Constant_x_l_08c9e/1 -> Product_3c439/2
  Add_75f47/1 -> Subtract_96906/1
  State_psi_d_SG_D_3_355d2/1 -> Add_75f47/2
  Product_3c439/1 -> Add_424ea/1
  Constant_x_qdd_03902/1 -> Subtract_278eb/2
  Add_c136d/1 -> Product_65876/2
  Constant_x_qdd_7b39c/1 -> Add_424ea/2
  State_psi_q_SG_D_3_d7233/1 -> Product_033c4/1
  Constant_x_l_c4f31/1 -> Product_8dcb6/2
  Subtract_64596/1 -> Divide_57be3/2
  Constant_x_l_7e92c/1 -> Subtract_ff6a0/2
  Constant_x_qd_d77c2/1 -> Subtract_278eb/1
  Constant_-1_bafa8/1 -> Product_6f939/1
  Subtract_3acb7/1 -> Divide_6a35a/2
  Constant_x_l_49bee/1 -> Product_6f939/2
  Product_ae869/1 -> Divide_6a35a/1
  Constant_-1_e3bfe/1 -> Product_f9b9c/1
  Product_f9b9c/1 -> Product_ae869/1
  Constant_x_dd_9d528/1 -> Subtract_bf7b9/1
  Constant_x_ddd_fc21e/1 -> Subtract_bf7b9/2
  Add_c8d7c/1 -> Blockout_T_e_SG_D_3_5900b/1
  State_psi_gq_SG_D_3_1cc94/1 -> Product_0aa49/1
  Product_033c4/1 -> Divide_a7e4b/1
  Add_424ea/1 -> Product_0aa49/2
  State_psi_fd_SG_D_3_44178/1 -> Product_fb25b/1
  Product_8dcb6/1 -> Add_38c6f/1
  Constant_x_qd_5fe02/1 -> Add_38c6f/2
  Constant_x_dd_3fcde/1 -> Subtract_3acb7/1
  State_psi_kq_SG_D_3_f2804/1 -> Product_06a99/1
  Constant_x_dd_c5962/1 -> Subtract_64596/1
  Subtract_278eb/1 -> Product_06a99/2
  Product_65876/1 -> Divide_7ca07/1
  Product_6f939/1 -> Add_d6943/1
  Add_38c6f/1 -> Divide_5f4e1/2
  Constant_x_qd_46c4d/1 -> Add_d6943/2
  Subtract_bf7b9/1 -> Product_ae869/2
  Constant_x_l_d57e3/1 -> Subtract_3acb7/2
  Constant_x_ddd_f9c1b/1 -> Subtract_ff6a0/1
  Product_0aa49/1 -> Divide_5f4e1/1
  Product_06a99/1 -> Divide_bf5f0/1
  Add_d6943/1 -> Divide_bf5f0/2
  Constant_x_ddd_03e8c/1 -> Divide_a7e4b/2
  Subtract_ff6a0/1 -> Product_fb25b/2
  Divide_5f4e1/1 -> Subtract_5e39d/1
  Constant_x_l_1b50a/1 -> Subtract_64596/2
  Divide_bf5f0/1 -> Subtract_5e39d/2
  Divide_6a35a/1 -> Add_75f47/1
  Product_fb25b/1 -> Divide_57be3/1
  Constant_-1_54cd6/1 -> Product_60f0d/1
  State_psi_d_SG_D_3_0515e/1 -> Product_60f0d/2
  Subtract_5e39d/1 -> Add_c136d/1
  Divide_57be3/1 -> Subtract_96906/2
  Product_60f0d/1 -> Product_65876/1
  Constant_x_qdd_35d62/1 -> Divide_7ca07/2
  Divide_7ca07/1 -> Add_c8d7c/1
  Divide_a7e4b/1 -> Add_c8d7c/2

== system case5/SG_D_3/d_E_fd_SG_D_3_block ==
  note: d_E_fd_SG_D_3 in case5
      | $\frac{V_{f,\mathrm{SG},D,3}-E_{\mathrm{fd},\mathrm{SG},D,3}\,K_{E}}{T_{E}}$
      | Automatically generated on 2025-10-31 19:13:05 .
  State_E_fd_SG_D_3_d3096 : Inport
  State_V_f_SG_D_3_2af07 : Inport  Port=2
  Add_f6eb9 : Sum
  Constant_-1_7b105 : Constant  Value=-1
  Constant_K_E_4a638 : Constant  Value=K_E
  Constant_T_E_77741 : Constant  Value=T_E
  Divide_9e3ea : Product  Inputs=*/
  Product_e1ea8 : Product
  Product_fa51f : Product
  Blockout_d_E_fd_SG_D_3_8336f : Outport
  wires:
  State_V_f_SG_D_3_2af07/1 -> Add_f6eb9/2
  Constant_-1_7b105/1 -> Product_fa51f/1
  State_E_fd_SG_D_3_d3096/1 -> Product_fa51f/2
  Constant_T_E_77741/1 -> Divide_9e3ea/2
  Product_fa51f/1 -> Product_e1ea8/1
  Product_e1ea8/1 -> Add_f6eb9/1
  Constant_K_E_4a638/1 -> Product_e1ea8/2
  Divide_9e3ea/1 -> Blockout_d_E_fd_SG_D_3_8336f/1
  Add_f6eb9/1 -> Divide_9e3ea/1

== system case5/SG_D_3/d_Px_1_SG_D_3_block ==
  note: d_Px_1_SG_D_3 in case5
      | $\frac{w_{\mathrm{SG},D,3}-2\,\pi \,f_{0}}{T_{w}}-\frac{\mathrm{Px}_{1,\mathrm{SG},D,3}}{T_{w}}$
      | Automatically generated on 2025-10-31 19:13:06 .
  State_Px_1_SG_D_3_e9303 : Inport
  State_w_SG_D_3_220ce : Inport  Port=2
  Add_1532a : Sum
  Add_7643b : Sum
  Constant_-1_7694c : Constant  Value=-1
  Constant_-2.0_e5ec0 : Constant  Value=-2.0
  Constant_T_w_654b1 : Constant  Value=T_w
  Constant_T_w_f2c52 : Constant  Value=T_w
  Constant_f0_7eaa7 : Constant  Value=f0
  Constant_pi_34ff6 : Constant  Value=pi
  Divide_31362 : Product  Inputs=*/
  Divide_eedfa : Product  Inputs=*/
  Product_67b16 : Product
  Product_c4af4 : Product
  Product_f4040 : Product
  Blockout_d_Px_1_SG_D_3_9be4e : Outport
  wires:
  Constant_f0_7eaa7/1 -> Product_f4040/2
  Constant_-1_7694c/1 -> Product_c4af4/1
  Constant_-2.0_e5ec0/1 -> Product_67b16/1
  Constant_pi_34ff6/1 -> Product_67b16/2
  Product_67b16/1 -> Product_f4040/1
  State_w_SG_D_3_220ce/1 -> Add_7643b/2
  Divide_31362/1 -> Add_1532a/1
  State_Px_1_SG_D_3_e9303/1 -> Product_c4af4/2
  Product_f4040/1 -> Add_7643b/1
  Product_c4af4/1 -> Divide_31362/1
  Constant_T_w_654b1/1 -> Divide_31362/2
  Add_7643b/1 -> Divide_eedfa/1
  Constant_T_w_f2c52/1 -> Divide_eedfa/2
  Divide_eedfa/1 -> Add_1532a/2
  Add_1532a/1 -> Blockout_d_Px_1_SG_D_3_9be4e/1

== system case5/SG_D_3/d_Px_2_SG_D_3_block ==
  note: d_Px_2_SG_D_3 in case5
      | $\frac{\mathrm{Px}_{1,\mathrm{SG},D,3}-T_{2}\,\left(\frac{\mathrm{Px}_{1,\mathrm{SG},D,3}}{T_{w}}-\frac{w_{\mathrm{SG},D,3}-2\,\pi \,f_{0}}{T_{w}}\right)}{T_{1}}-\frac{\mathrm{Px}_{2,\mathrm{SG},D,3}}{T_{1}}$
      | Automatically generated on 2025-10-31 19:13:08 .
  State_Px_2_SG_D_3_b50b4 : Inport
  State_Px_1_SG_D_3_ebea2 : Inport  Port=2
  State_Px_1_SG_D_3_6c166 : Inport  Port=3
  State_w_SG_D_3_ac5cc : Inport  Port=4
  Add_0b2ef : Sum
  Add_48cb7 : Sum
  Add_585c8 : Sum
  Add_ce93c : Sum
  Constant_-1_d0b5a : Constant  Value=-1
  Constant_-1_e1227 : Constant  Value=-1
  Constant_-2.0_0d266 : Constant  Value=-2.0
  Constant_T_1_840e8 : Constant  Value=T_1
  Constant_T_1_86657 : Constant  Value=T_1
  Constant_T_2_7158d : Constant  Value=T_2
  Constant_T_w_99f80 : Constant  Value=T_w
  Constant_T_w_a06f4 : Constant  Value=T_w
  Constant_f0_0e999 : Constant  Value=f0
  Constant_pi_6116d : Constant  Value=pi
  Divide_303ac : Product  Inputs=*/
  Divide_4113e : Product  Inputs=*/
  Divide_81526 : Product  Inputs=*/
  Divide_bc8dc : Product  Inputs=*/
  Product_04509 : Product
  Product_071b2 : Product
  Product_0ef70 : Product
  Product_3d0c8 : Product
  Product_54167 : Product
  Blockout_d_Px_2_SG_D_3_d6435 : Outport
  wires:
  State_Px_1_SG_D_3_6c166/1 -> Product_04509/2
  Constant_-2.0_0d266/1 -> Product_3d0c8/1
  Constant_f0_0e999/1 -> Product_071b2/2
  Constant_pi_6116d/1 -> Product_3d0c8/2
  Product_3d0c8/1 -> Product_071b2/1
  State_w_SG_D_3_ac5cc/1 -> Add_48cb7/2
  Constant_-1_d0b5a/1 -> Product_04509/1
  Product_071b2/1 -> Add_48cb7/1
  Product_04509/1 -> Divide_303ac/1
  Constant_T_w_99f80/1 -> Divide_303ac/2
  Add_48cb7/1 -> Divide_4113e/1
  Constant_T_w_a06f4/1 -> Divide_4113e/2
  Divide_303ac/1 -> Add_ce93c/1
  Divide_4113e/1 -> Add_ce93c/2
  Constant_T_2_7158d/1 -> Product_0ef70/1
  Add_ce93c/1 -> Product_0ef70/2
  Constant_-1_e1227/1 -> Product_54167/1
  Product_0ef70/1 -> Add_0b2ef/2
  State_Px_2_SG_D_3_b50b4/1 -> Product_54167/2
  State_Px_1_SG_D_3_ebea2/1 -> Add_0b2ef/1
  Product_54167/1 -> Divide_bc8dc/1
  Add_585c8/1 -> Blockout_d_Px_2_SG_D_3_d6435/1
  Constant_T_1_840e8/1 -> Divide_bc8dc/2
  Add_0b2ef/1 -> Divide_81526/1
  Constant_T_1_86657/1 -> Divide_81526/2
  Divide_bc8dc/1 -> Add_585c8/1
  Divide_81526/1 -> Add_585c8/2

== system case5/SG_D_3/d_Px_3_SG_D_3_block ==
  note: d_Px_3_SG_D_3 in case5
      | $\frac{\mathrm{Px}_{2,\mathrm{SG},D,3}+T_{4}\,\left(\frac{\mathrm{Px}_{1,\mathrm{SG},D,3}-T_{2}\,\left(\frac{\mathrm{Px}_{1,\mathrm{SG},D,3}}{T_{w}}-\frac{w_{\mathrm{SG},D,3}-2\,\pi \,f_{0}}{T_{w}}\right)}{T_{1}}-\frac{\mathrm{Px}_{2,\mathrm{SG},D,3}}{T_{1}}\right)}{T_{3}}-\frac{\mathrm{Px}_{3,\mathrm{SG},D,3}}{T_{3}}$
      | Automatically generated on 2025-10-31 19:13:11 .
  State_Px_3_SG_D_3_2f57b : Inport
  State_Px_2_SG_D_3_8f252 : Inport  Port=2
  State_Px_2_SG_D_3_5d3da : Inport  Port=3
  State_Px_1_SG_D_3_769ed : Inport  Port=4
  State_Px_1_SG_D_3_ab3a0 : Inport  Port=5
  State_w_SG_D_3_03b1d : Inport  Port=6
  Add_150a0 : Sum
  Add_4d367 : Sum
  Add_74b05 : Sum
  Add_a6466 : Sum
  Add_c1950 : Sum
  Add_e8b9b : Sum
  Constant_-1_5cbb3 : Constant  Value=-1
  Constant_-1_6b6e6 : Constant  Value=-1
  Constant_-1_dd8f2 : Constant  Value=-1
  Constant_-2.0_09ece : Constant  Value=-2.0
  Constant_T_1_319a3 : Constant  Value=T_1
  Constant_T_1_d32d0 : Constant  Value=T_1
  Constant_T_2_2988e : Constant  Value=T_2
  Constant_T_3_f2ded : Constant  Value=T_3
  Constant_T_3_fb91b : Constant  Value=T_3
  Constant_T_4_69b7d : Constant  Value=T_4
  Constant_T_w_2a5fe : Constant  Value=T_w
  Constant_T_w_d1d0f : Constant  Value=T_w
  Constant_f0_f0395 : Constant  Value=f0
  Constant_pi_af87c : Constant  Value=pi
  Divide_2c5c6 : Product  Inputs=*/
  Divide_4e427 : Product  Inputs=*/
  Divide_55294 : Product  Inputs=*/
  Divide_7d519 : Product  Inputs=*/
  Divide_85ae3 : Product  Inputs=*/
  Divide_c6641 : Product  Inputs=*/
  Product_058b3 : Product
  Product_0e3b2 : Product
  Product_7b591 : Product
  Product_85bee : Product
  Product_b83a9 : Product
  Product_c2781 : Product
  Product_d5e82 : Product
  Blockout_d_Px_3_SG_D_3_07f5b : Outport
  wires:
  State_Px_1_SG_D_3_ab3a0/1 -> Product_d5e82/2
  Constant_f0_f0395/1 -> Product_7b591/2
  Constant_-2.0_09ece/1 -> Product_85bee/1
  Add_74b05/1 -> Divide_4e427/1
  Constant_pi_af87c/1 -> Product_85bee/2
  Product_85bee/1 -> Product_7b591/1
  State_w_SG_D_3_03b1d/1 -> Add_c1950/2
  Constant_T_w_d1d0f/1 -> Divide_7d519/2
  Constant_-1_6b6e6/1 -> Product_d5e82/1
  Product_7b591/1 -> Add_c1950/1
  Product_d5e82/1 -> Divide_7d519/1
  Add_c1950/1 -> Divide_c6641/1
  Product_c2781/1 -> Divide_85ae3/1
  Constant_T_w_2a5fe/1 -> Divide_c6641/2
  Divide_7d519/1 -> Add_e8b9b/1
  Divide_c6641/1 -> Add_e8b9b/2
  Constant_T_2_2988e/1 -> Product_0e3b2/1
  Add_e8b9b/1 -> Product_0e3b2/2
  Constant_-1_5cbb3/1 -> Product_c2781/1
  State_Px_2_SG_D_3_5d3da/1 -> Product_c2781/2
  State_Px_1_SG_D_3_769ed/1 -> Add_74b05/1
  Constant_T_3_fb91b/1 -> Divide_55294/2
  Product_0e3b2/1 -> Add_74b05/2
  Constant_T_1_d32d0/1 -> Divide_85ae3/2
  Add_150a0/1 -> Product_b83a9/2
  Constant_T_1_319a3/1 -> Divide_4e427/2
  Divide_2c5c6/1 -> Add_a6466/2
  Divide_85ae3/1 -> Add_150a0/1
  Divide_4e427/1 -> Add_150a0/2
  Constant_T_4_69b7d/1 -> Product_b83a9/1
  Constant_-1_dd8f2/1 -> Product_058b3/1
  State_Px_3_SG_D_3_2f57b/1 -> Product_058b3/2
  State_Px_2_SG_D_3_8f252/1 -> Add_4d367/1
  Product_b83a9/1 -> Add_4d367/2
  Product_058b3/1 -> Divide_55294/1
  Add_4d367/1 -> Divide_2c5c6/1
  Constant_T_3_f2ded/1 -> Divide_2c5c6/2
  Divide_55294/1 -> Add_a6466/1
  Add_a6466/1 -> Blockout_d_Px_3_SG_D_3_07f5b/1
